simulink model "assignment"  (R2018b)
settings: Solver=VariableStepAuto  StartTime=0.0  StopTime=50  RelTol=1e-3
libraries: cstblocks x1
settings Model: Creator=FARYAL  LastModifiedBy=FARYAL

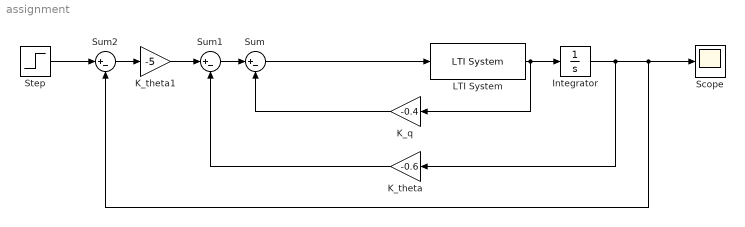
== system assignment ==
  Integrator : Integrator
  "K_q " : Gain  Gain=-0.4
  K_theta : Gain  Gain=-0.6
  K_theta1 : Gain  Gain=-5
  LTI System : cstblocks/LTI System  sys=tf([-182.4 -99.72 -1.148 0],[1 1.262 8.134 0.01107 -0.01284])  IC=[]
  Scope : Scope
  Step : Step  Before=1  SampleTime=0
  Sum : Sum  Inputs=|+-
  Sum1 : Sum  Inputs=|+-
  Sum2 : Sum  Inputs=|+-
  wires:
  Sum/1 -> LTI System/1
  "K_q "/1 -> Sum/2
  LTI System/1 -> "K_q "/1, Integrator/1
  Integrator/1 -> Scope/1, Sum2/2, K_theta/1
  K_theta/1 -> Sum1/2
  Sum2/1 -> K_theta1/1
  Step/1 -> Sum2/1
  Sum1/1 -> Sum/1
  K_theta1/1 -> Sum1/1
